simulink model "motor_control_encoder_part_A"  (R2023b)
settings: Solver=ode3  StartTime=0.0  StopTime=45  FixedStep=0.01  RelTol=1e-3  EnableMultiTasking=on
libraries: arduinolib x6
settings Model: FPTRunName=Active  ExtModeTrigDuration=2  Creator=joshuayoo  LastModifiedBy=patel
settings SolverCC: AlgebraicLoopSolver=TrustRegion  AutoInsertRateTranBlk=on
settings DataIOCC: LimitDataPoints=on  SaveFormat=Array
settings OptimizationCC: ReuseModelBlockBuffer=off  ExpressionDepthLimit=2147483647  LifeSpan=Inf  MaxStackSize=64
settings DebuggingCC: UnderspecifiedInitializationDetection=Classic  MergeDetectMultiDrivingBlocksExec=none  FcnCallInpInsideContextMsg=warning  UnconnectedInputMsg=warning  UnconnectedOutputMsg=warning  UnconnectedLineMsg=warning  AllowSymbolicDim=off  StateNameClashWarn=warning  SFUnexpectedBacktrackingDiag=warning  SFNoUnconditionalDefaultTransitionDiag=warning  SFExecutionAtInitializationDiag=none  ArithmeticOperatorsInVariantConditions=warning
settings HardwareCC: ProdBitPerInt=16  ProdBitPerPointer=16  ProdBitPerSizeT=16  ProdBitPerPtrDiffT=16  ProdLargestAtomicFloat=None  ProdWordSize=8  ProdHWDeviceType=Atmel->AVR  UseEmbeddedCoderFeatures=off  UseSimulinkCoderFeatures=off
settings ModelReferenceCC: EnableRefExpFcnMdlSchedulingChecks=on  PropagateSignalLabelsOutOfModel=off
settings SFSimCC: SimUseLocalCustomCode=off  CustomCodeUndefinedFunction=UseInterfaceOnly
settings RTWCC: Description=Embedded Coder  SystemTargetFile=ert.tlc  HardwareBoard=Arduino Uno  TemplateMakefile=ert_default_tmf  GenerateReport=on  RTWVerbose=off  RTWUseLocalCustomCode=off  Toolchain=Arduino AVR  BuildConfiguration=Faster Runs  LaunchReport=on
settings CodeAppCC: ForceParamTrailComments=on  OperatorAnnotations=on  MangleLength=10  StateflowObjectComments=on  MATLABSourceComments=on
settings ERTTargetCC: MultiwordLength=2048  ERTCustomFileBanners=off  SupportContinuousTime=on  SupportNonInlinedSFcns=on  RemoveResetFunc=off  SupportVariableSizeSignals=on  ModelStepFunctionPrototypeControlCompliant=off  ExtModeTransport=3  ExtModeStaticAlloc=on  ExtModeAutomaticAllocSize=off  ExtModeStaticAllocSize=250  ExtModeMexFile=ext_xcp  ExtModeIntrfLevel=Level2 - Open
settings ConfigComp: CovMetricSettings=dw  CovSaveCumulativeToWorkspaceVar=on  CovSaveSingleToWorkspaceVar=on  CovExternalEMLEnable=off  CovSFcnEnable=off

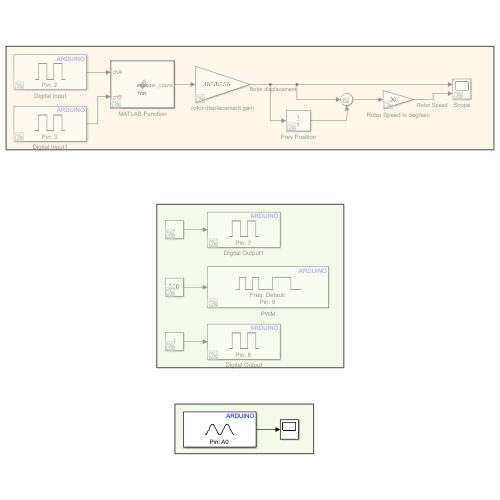
[thumbnail: Simulink's stored preview of the top-level diagram]
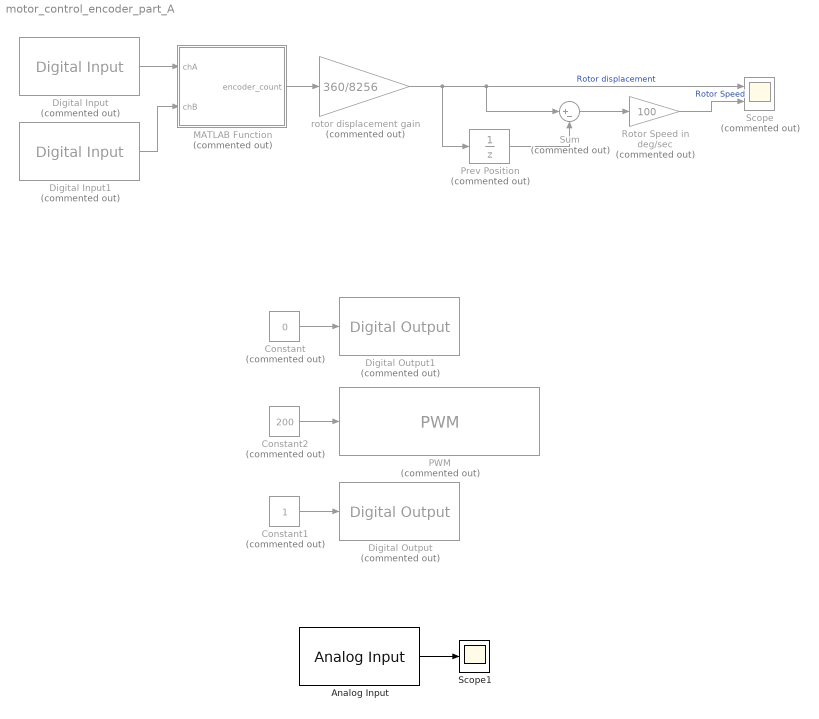
== system motor_control_encoder_part_A ==
  Analog Input : arduinolib/Analog Input  pinNumber=0  ReadResultsOnly=off  ConversionTriggerSource=Software  ExternalTriggerType=uint32( 0 )  OutputDataType=uint16  EnableConversionCompleteNotify=off  EnableOuputStatus=off  SampleTime=-1  blockPlatform=arduino
  Constant : Constant  Commented=on  Value=0
  Constant1 : Constant  Commented=on
  Constant2 : Constant  Commented=on  Value=200
  Digital Input : arduinolib/Digital Input  Commented=on  pinNumber=2  mode=Default  Direction=input  SampleTime=0.1  blockPlatform=arduino
  Digital Input1 : arduinolib/Digital Input  Commented=on  pinNumber=3  mode=Default  Direction=input  SampleTime=0.1  blockPlatform=arduino
  Digital Output : arduinolib/Digital Output  Commented=on  pinNumber=8  Direction=output  blockPlatform=arduino
  Digital Output1 : arduinolib/Digital Output  Commented=on  pinNumber=7  Direction=output  blockPlatform=arduino
  MATLAB Function : MATLAB Function  Commented=on  TreatAsAtomicUnit=on
  PWM : arduinolib/PWM  Commented=on  pinNumber=9  frequencyType=Default  desiredFrequency=490.2  achievableFrequency=490.2
  Prev Position : UnitDelay  Commented=on  SampleTime=-1  HasFrameUpgradeWarning=on
  Rotor Speed in deg/sec : Gain  Commented=on  Gain=100
  Scope : Scope  Commented=on  NumInputPorts=2
  Scope1 : Scope
  Sum : Sum  Commented=on  Inputs=|+-
  rotor displacement gain : Gain  Commented=on  Gain=360/8256
  wires:
  Constant/1 -> Digital Output1/1
  MATLAB Function/1(encoder_count) -> rotor displacement gain/1
  Constant1/1 -> Digital Output/1
  Constant2/1 -> PWM/1
  Analog Input/1 -> Scope1/1
  rotor displacement gain/1 -> Scope/1, Sum/1, Prev Position/1  "Rotor displacement"
  Rotor Speed in deg/sec/1 -> Scope/2  "Rotor Speed"
  Digital Input1/1 -> MATLAB Function/2(chB)
  Digital Input/1 -> MATLAB Function/1(chA)
  Prev Position/1 -> Sum/2
  Sum/1 -> Rotor Speed in deg/sec/1

== matlab function motor_control_encoder_part_A/MATLAB Function ==
  data: chA input; encoder_count output; chB input
function encoder_count = fcn(chA, chB)

persistent count last_state;

if isempty(count)
    count = 0;
    last_state = [0, 0];
end

current_state = double([chA, chB]);

% This lookup table determines the change in count (+1, -1, or 0)
% based on the transition from the last state to the current state.
% Rows are the last state [A,B]: 00, 01, 11, 10
% Columns are the current state [A,B]: 00, 01, 11, 10
state_table = [ 0, -1,  1,  0;  % Last state was 00
                1,  0,  0, -1;  % Last state was 01
               -1,  0,  0,  1;  % Last state was 11
                0,  1, -1,  0]; % Last state was 10

% convert the binary states to decimal indices for the table
last_idx = last_state(1) * 2 + last_state(2) + 1;
current_idx = current_state(1) * 2 + current_state(2) + 1;

% update the count based on the state transition
increment = state_table(last_idx, current_idx);
count = count + increment;

% save the current state for the next time step
last_state = current_state;

encoder_count = count;
